simulink model "ball_drop"  (Simulink 6.6)
settings: Solver=FixedStepDiscrete  SolverMode=SingleTasking  StartTime=0.0  StopTime=Inf  FixedStep=.001  RelTol=1e-3
libraries: xpclib x6, xpcnilib x5, limblab x2, simulink x1
settings Model: Creator=Selket  LastModifiedBy=Selket  BufferReuse=off  ProdHWDeviceType=32-bit xPC Target (Intel Pentium)
settings OptimizationCC: BlockReduction=off  OptimizeBlockIOStorage=off  BufferReuse=off  ExpressionFolding=off  LocalBlockOutputs=off
settings HardwareCC: ProdIntDivRoundTo=Zero  ProdEndianess=LittleEndian  ProdHWDeviceType=32-bit xPC Target (Intel Pentium)
settings RTWCC: SystemTargetFile=xpctarget.tlc  TemplateMakefile=xpc_default_tmf  Description=xPC Target  ProcessScript=xpctarget_make_rtw_hook
settings xpcTargetCC: TargetFcnLib=ansi_tfl_tmw.mat  GenFloatMathFcnCalls=ANSI_C  PortableWordSizes=off  xPCisDownloadable=off
settings CustomProperty: DataType=string

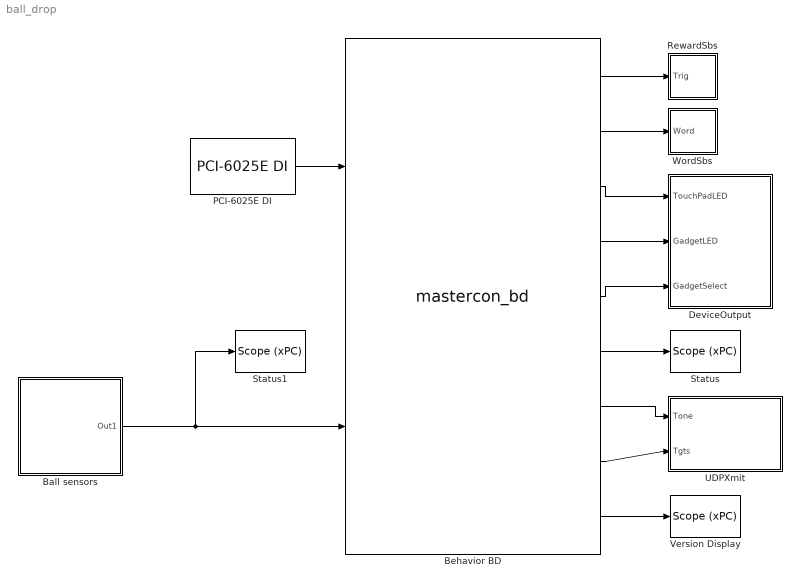
== system ball_drop ==
  Ball sensors : Subsystem
  Behavior BD : S-Function  FunctionName=mastercon_bd  Parameters=1 2 3 4 5 6 7 8 9
      mask Display:
      | disp('Master Control\nBall-Drop')
      | port_label('input',1,'touch pad')
      | port_label('input',2,'ball sensors')
      | port_label('output',1,'Reward')
      | port_label('output',2,'Word')
      | port_label('output',3,'TP LED')
      | port_label('output',4,'Gadget LED')
      | port_label('output',5,'Gadget Select')
      | port_label('output',6,'Status')
      | port_label('output',7,'Tone')
      | port_label('output',8,'Targets')
      | port_label('output',9,'Version')
  DeviceOutput : Subsystem
  PCI-6025E DI : xpcnilib/Digital Input/PCI-6025E DI  channel=[3]  sampletime=0.001  slot=-1
  RewardSbs : Subsystem
  Status : xpclib/Misc./Scope (xPC)   SystemSampleTime=-1  scopeno=1  scopetype=Target  autostart=on  viewmode=Numerical  formatstr='%6.0f State,%6.0f Rewards,%6.0f Aborts,%6.0f Failures'  grid=on  ylimits=[-10,10]  nosamples=10  noprepostsamples=0  interleave=10  triggermode=FreeRun  triggersignal=1  triggerlevel=0.0  triggerslope=Either  triggerscope=1  triggersample=0  filename=data.dat  mode=Lazy  writesize=512  autorestart=off
  Status1 : xpclib/Misc./Scope (xPC)   SystemSampleTime=-1  scopeno=2  scopetype=Target  autostart=on  viewmode=Numerical  formatstr=' %6.6f X, %6.6f Y'  grid=on  ylimits=[-10,10]  nosamples=10  noprepostsamples=0  interleave=10  triggermode=FreeRun  triggersignal=1  triggerlevel=0.0  triggerslope=Either  triggerscope=1  triggersample=0  filename=data.dat  mode=Lazy  writesize=512  autorestart=off
  UDPXmit : Subsystem
  Version Display : xpclib/Misc./Scope (xPC)   SystemSampleTime=-1  scopeno=3  scopetype=Target  autostart=on  viewmode=Numerical  formatstr='%6.0f major,%6.0f minor,%6.0f revision,%6.0f build'  grid=on  ylimits=[-10,10]  nosamples=10  noprepostsamples=0  interleave=10  triggermode=FreeRun  triggersignal=1  triggerlevel=0.0  triggerslope=Either  triggerscope=1  triggersample=0  filename=data.dat  mode=Lazy  writesize=512  autorestart=off
  WordSbs : Subsystem
  wires:
  Behavior BD/2 -> WordSbs/1(Word)
  Behavior BD/3 -> DeviceOutput/1(TouchPadLED)
  Behavior BD/4 -> DeviceOutput/2(GadgetLED)
  Behavior BD/5 -> DeviceOutput/3(GadgetSelect)
  Behavior BD/6 -> Status/1
  Behavior BD/1 -> RewardSbs/1(Trig)
  Behavior BD/8 -> UDPXmit/2(Tgts)
  PCI-6025E DI/1 -> Behavior BD/1
  Ball sensors/1(Out1) -> Behavior BD/2, Status1/1
  Behavior BD/7 -> UDPXmit/1(Tone)
  Behavior BD/9 -> Version Display/1

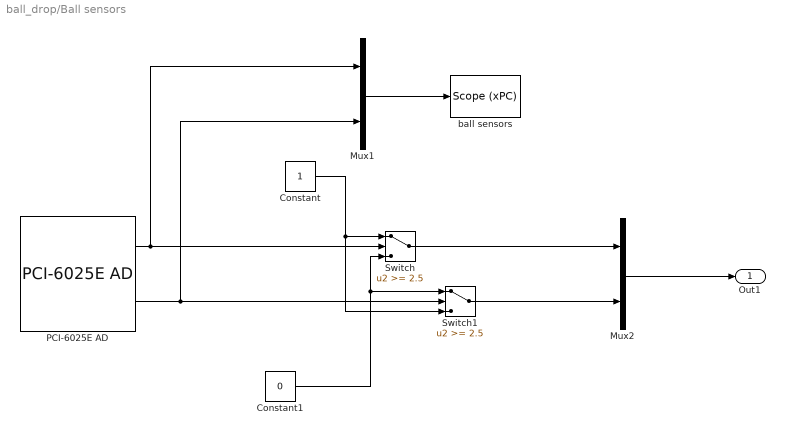
== system ball_drop/Ball sensors ==
  Constant : Constant
  Constant1 : Constant  Value=0
  Mux1 : Mux  Inputs=2
  Mux2 : Mux  Inputs=2
  PCI-6025E AD : xpcnilib/A//D/PCI-6025E AD  channel=[9 10]  range=[-10]  coupling=[0]  sampletime=0.001  slot=-1
  Switch : Switch  Threshold=2.5
  Switch1 : Switch  Threshold=2.5
  ball sensors : xpclib/Misc./Scope (xPC)   SystemSampleTime=-1  scopeno=4  scopetype=Target  autostart=on  viewmode=Numerical  formatstr=' %2.2f Pick up, %2.2f drop'  grid=on  ylimits=[-10,10]  nosamples=10  noprepostsamples=0  interleave=10  triggermode=FreeRun  triggersignal=1  triggerlevel=0.0  triggerslope=Either  triggerscope=1  triggersample=0  filename=data.dat  mode=Lazy  writesize=512  autorestart=off
  Out1 : Outport
  wires:
  PCI-6025E AD/1 -> Mux1/1, Switch/2
  PCI-6025E AD/2 -> Mux1/2, Switch1/2
  Mux1/1 -> ball sensors/1
  Constant/1 -> Switch/1, Switch1/3
  Constant1/1 -> Switch/3, Switch1/1
  Switch/1 -> Mux2/1
  Switch1/1 -> Mux2/2
  Mux2/1 -> Out1/1

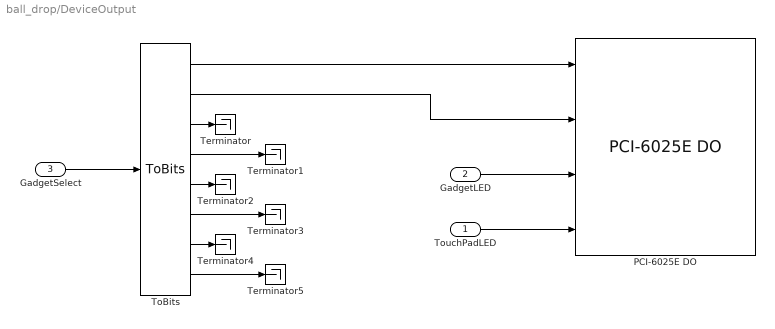
== system ball_drop/DeviceOutput ==
  TouchPadLED : Inport
  GadgetLED : Inport  Port=2
  GadgetSelect : Inport  Port=3
  PCI-6025E DO : xpcnilib/Digital Output/PCI-6025E DO  channel=[4 5 6 8]  reset=[1]  initValue=[0]  sampletime=0.001  slot=-1
  Terminator{,1..5} (6 alike) : Terminator
  ToBits : limblab/ToBits
  wires:
  GadgetLED/1 -> PCI-6025E DO/3
  TouchPadLED/1 -> PCI-6025E DO/4
  GadgetSelect/1 -> ToBits/1
  ToBits/1 -> PCI-6025E DO/1
  ToBits/2 -> PCI-6025E DO/2
  ToBits/4 -> Terminator1/1
  ToBits/3 -> Terminator/1
  ToBits/5 -> Terminator2/1
  ToBits/6 -> Terminator3/1
  ToBits/7 -> Terminator4/1
  ToBits/8 -> Terminator5/1

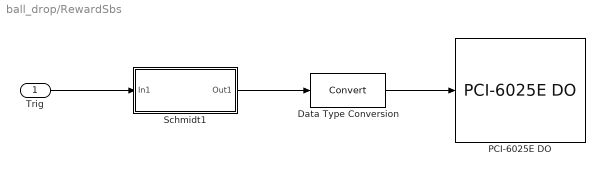
== system ball_drop/RewardSbs ==
  Trig : Inport
  Data Type Conversion : DataTypeConversion
  PCI-6025E DO : xpcnilib/Digital Output/PCI-6025E DO  channel=[2]  reset=[1]  initValue=[0]  sampletime=0.001  slot=-1
  Schmidt1 : Subsystem  mask(Schmidt Trigger){Time=.3}
      mask help: Creates an output pulse of the specified time in seconds when trig goes high
      mask Help: Creates an output pulse of the specified time in seconds when trig goes high
      mask Display:
      | port_label('output',1,'out')
      | port_label('input',1,'trig')
      | fprintf('t = %.2f',Time)
  wires:
  Trig/1 -> Schmidt1/1(In1)
  Data Type Conversion/1 -> PCI-6025E DO/1
  Schmidt1/1(Out1) -> Data Type Conversion/1

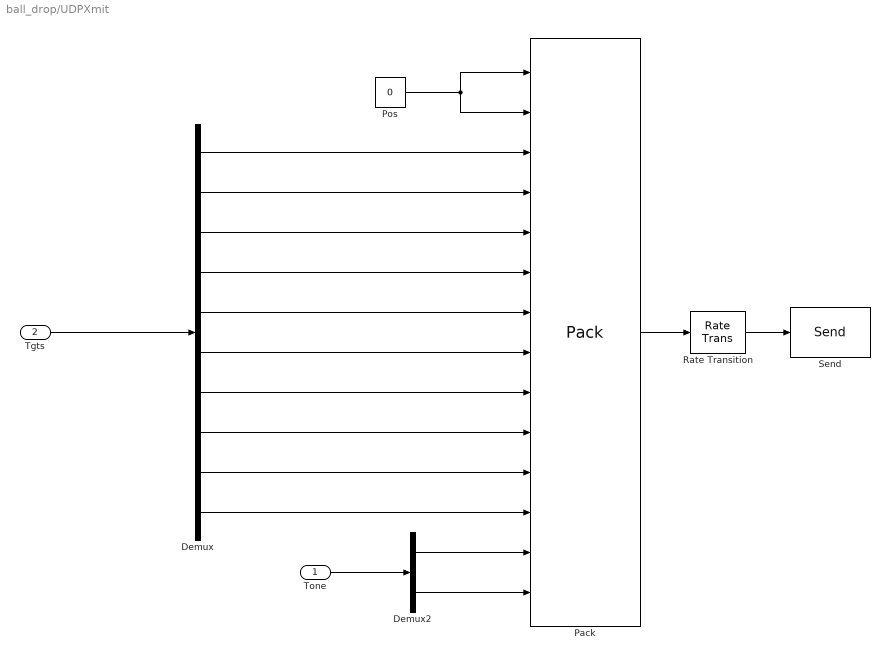
== system ball_drop/UDPXmit ==
  Tone : Inport
  Tgts : Inport  Port=2
  Demux : Demux  Outputs=10
  Demux2 : Demux  Outputs=2
  Pack : xpclib/UDP/Pack  datatypes={'double','double','double','double','double','double','double','double','double','double','double','double','double','double'}  byteAlign=1
  Pos : Constant  Value=0
  Rate Transition : RateTransition
  Send : xpclib/UDP/Send  ipAddress=192.168.0.2  ipPort=25000  localPort=-1  sampletime=.02
  wires:
  Rate Transition/1 -> Send/1
  Pack/1 -> Rate Transition/1
  Demux2/1 -> Pack/13
  Demux2/2 -> Pack/14
  Tone/1 -> Demux2/1
  Tgts/1 -> Demux/1
  Demux/3 -> Pack/5
  Demux/10 -> Pack/12
  Demux/9 -> Pack/11
  Demux/8 -> Pack/10
  Demux/7 -> Pack/9
  Demux/6 -> Pack/8
  Demux/5 -> Pack/7
  Demux/4 -> Pack/6
  Demux/2 -> Pack/4
  Demux/1 -> Pack/3
  Pos/1 -> Pack/1, Pack/2

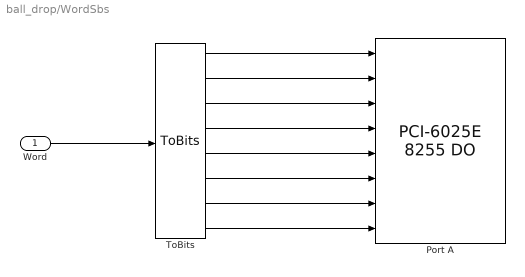
== system ball_drop/WordSbs ==
  Word : Inport
  Port A : xpcnilib/Digital Output/PCI-6025E 8255 DO  channel=1:8  port=A  reset=[1]  initValue=[0]  chip=1  sampletime=-1  slot=-1
  ToBits : limblab/ToBits
  wires:
  Word/1 -> ToBits/1
  ToBits/1 -> Port A/1
  ToBits/2 -> Port A/2
  ToBits/3 -> Port A/3
  ToBits/4 -> Port A/4
  ToBits/5 -> Port A/5
  ToBits/6 -> Port A/6
  ToBits/7 -> Port A/7
  ToBits/8 -> Port A/8

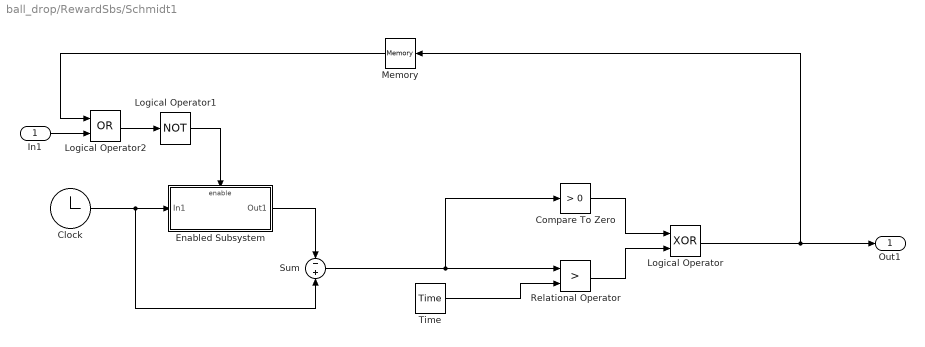
== system ball_drop/RewardSbs/Schmidt1 ==
  In1 : Inport
  Clock : Clock
  Compare To Zero : simulink/Logic and Bit Operations/Compare To Zero  SystemSampleTime=-1  relop=>  LogicOutDataTypeMode=uint8  ZeroCross=off
  Enabled Subsystem : Subsystem  TreatAsAtomicUnit=on
  Logical Operator : Logic  Operator=XOR  AllPortsSameDT=off  OutDataTypeMode=Boolean  SampleTime=.001
  Logical Operator1 : Logic  Operator=NOT  AllPortsSameDT=off  OutDataTypeMode=Boolean
  Logical Operator2 : Logic  Operator=OR  AllPortsSameDT=off  OutDataTypeMode=Boolean  SampleTime=.001
  Memory : Memory  Orientation=left
  Relational Operator : RelationalOperator  Operator=>  LogicOutDataTypeMode=Boolean
  Sum : Sum  Inputs=-+
  Time : Constant  Value=Time
  Out1 : Outport
  wires:
  Clock/1 -> Enabled Subsystem/1(In1), Sum/2
  Enabled Subsystem/1(Out1) -> Sum/1
  Sum/1 -> Compare To Zero/1, Relational Operator/1
  Time/1 -> Relational Operator/2
  Compare To Zero/1 -> Logical Operator/1
  Relational Operator/1 -> Logical Operator/2
  Logical Operator1/1 -> Enabled Subsystem/Enable
  Logical Operator/1 -> Out1/1, Memory/1
  In1/1 -> Logical Operator2/2
  Logical Operator2/1 -> Logical Operator1/1
  Memory/1 -> Logical Operator2/1

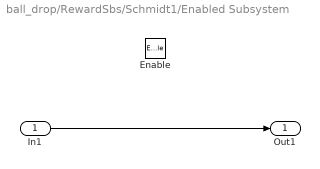
== system ball_drop/RewardSbs/Schmidt1/Enabled Subsystem ==
  In1 : Inport
  Enable : EnablePort
  Out1 : Outport
  wires:
  In1/1 -> Out1/1
